simulink model "Systeme"  (R2020a)
settings: Solver=VariableStepAuto  StartTime=0.0  StopTime=10.0  RelTol=1e-3
settings Model: Creator=Lamarre  LastModifiedBy=lamarre

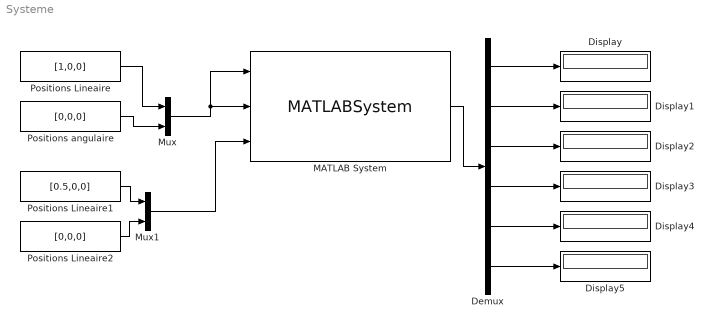
== system Systeme ==
  Demux : Demux  Outputs=6
  Display{,1..5} (6 alike) : Display
  MATLAB System : MATLABSystem  System=Modele_dinamique_AUV  SimulateUsing=Code generation
      mask Type: Modele_dinamique_AUV
      mask Display:
      | disp('Modele_dinamique_AUV');
      | port_label('input',1,'pos');
      | port_label('input',2,'vitesse');
      | port_label('input',3,'acc');
      | port_label('output',1,'Force');
  Mux : Mux  Inputs=2
  Mux1 : Mux  Inputs=2
  Positions Lineaire : Constant  Value=[1,0,0]
  Positions Lineaire1 : Constant  Value=[0.5,0,0]
  Positions Lineaire2 : Constant  Value=[0,0,0]
  Positions angulaire : Constant  Value=[0,0,0]
  wires:
  Demux/1 -> Display/1
  Demux/2 -> Display1/1
  Demux/3 -> Display2/1
  Demux/4 -> Display3/1
  Demux/5 -> Display4/1
  Demux/6 -> Display5/1
  Positions Lineaire/1 -> Mux/1
  Positions angulaire/1 -> Mux/2
  MATLAB System/1 -> Demux/1
  Mux/1 -> MATLAB System/1, MATLAB System/2
  Positions Lineaire2/1 -> Mux1/2
  Positions Lineaire1/1 -> Mux1/1
  Mux1/1 -> MATLAB System/3
